simulink model "StateDiagram3"  (R2025b)
settings: Solver=VariableStepAuto  StartTime=0.0  StopTime=Inf  RelTol=1e-3
libraries: simulink_extras x1
settings Model: Creator=Soochan Kim  LastModifiedBy=Soochan Kim

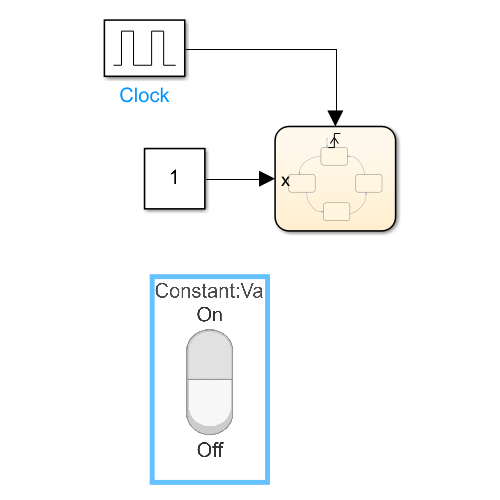
[thumbnail: Simulink's stored preview of the top-level diagram]
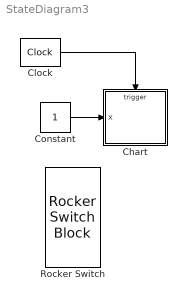
== system StateDiagram3 ==
  Chart : Stateflow chart  TreatAsAtomicUnit=on
  Clock : simulink_extras/Flip Flops/Clock  period=2
  Constant : Constant
  Rocker Switch : RockerSwitchBlock
  wires:
  Constant/1 -> Chart/1(x)
  Clock/1 -> Chart/Trigger

== stateflow chart StateDiagram3/Chart ==
  settings: executeAtInitialization=1
  state S0
  state S02
  state S01
  state S03
  (default) -> S0
  S01 -> S0 : [x==1]
  S0 -> S02 : [x==1]
  S02 -> S03 : [x==0]
  S03 -> S01 : [x==1]
  data: x input
  events: clk input RISING_EDGE_EVENT
